simulink model "lab1"  (R2018a)
settings: Solver=ode45  StartTime=0.0  StopTime=5.0  RelTol=1e-3
libraries: powerlib x1
settings Model: Creator=KJ_Fa  LastModifiedBy=KJ_Fa

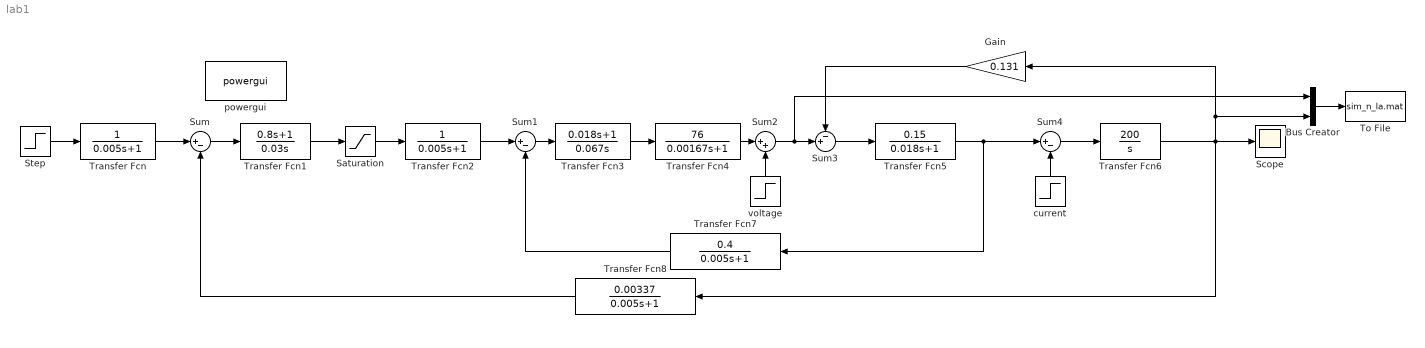
== system lab1 ==
  Bus Creator : BusCreator  Inputs=2
  Gain : Gain  Gain=0.131
  Saturation : Saturate  UpperLimit=8  LowerLimit=-8
  Scope : Scope
  Step : Step  Time=0  After=5  SampleTime=0
  Sum : Sum  Inputs=|+-
  Sum1 : Sum  Inputs=|+-
  Sum2 : Sum  Inputs=|++
  Sum3 : Sum  Inputs=-+|
  Sum4 : Sum  Inputs=|+-
  To File : ToFile  Filename=sim_n_la.mat  MatrixName=signals
  Transfer Fcn : TransferFcn  Denominator=[0.005 1]
  Transfer Fcn1 : TransferFcn  Numerator=[0.8 1]  Denominator=[0.03 0]
  Transfer Fcn2 : TransferFcn  Denominator=[0.005 1]
  Transfer Fcn3 : TransferFcn  Numerator=[0.018 1]  Denominator=[0.067 0]
  Transfer Fcn4 : TransferFcn  Numerator=[76]  Denominator=[0.00167 1]
  Transfer Fcn5 : TransferFcn  Numerator=[0.15]  Denominator=[0.018 1]
  Transfer Fcn6 : TransferFcn  Numerator=[200]  Denominator=[1 0]
  Transfer Fcn7 : TransferFcn  Numerator=[0.4]  Denominator=[0.005 1]
  Transfer Fcn8 : TransferFcn  Numerator=[0.00337]  Denominator=[0.005 1]
  current : Step  Time=3.5  After=0  SampleTime=0
  powergui : powerlib/powergui  Priority=1  SimulationMode=Continuous  SampleTime=50e-6  frequency=60  Iterations=50  frequencyindice=60  Pbase=100e6  ErrMax=1e-4  UnitsV=kV  UnitsW=MW  buscounter=0  FunctionMessages=off  echomessages=off  EnableUseOfTLC=off  CurrentSourceSwitches=off  DisableSnubberDevices=off  DisableRonSwitches=off  DisableVfSwitches=off  DisplayEquations=off  SolverType=Tustin/Backward Euler (TBE)  Interpol=off  ExternalGateDelay=off  methode=off  Ts=100  x0status=blocks  SPID=on  SwTol=0  HookPort=off  RestoreLinks=warning  ResistiveCurrentMeasurement=off  Frange=[0:2:500]  Ylog=off  Xlog=on  ShowGrid=off  save=off  variable=ZData  structure=0  ZoomFFT=off  StartTime=0.0  cycles=1  DisplayStyle=1  fundamental=60  FreqAxis=off  MaxFrequency=1000  frequencyindicesteady=1  RmsSteady=1  display=off
  voltage : Step  Time=3.5  After=-100  SampleTime=0
  wires:
  Step/1 -> Transfer Fcn/1
  Transfer Fcn/1 -> Sum/1
  Sum/1 -> Transfer Fcn1/1
  Transfer Fcn1/1 -> Saturation/1
  Saturation/1 -> Transfer Fcn2/1
  Transfer Fcn2/1 -> Sum1/1
  Sum1/1 -> Transfer Fcn3/1
  Transfer Fcn3/1 -> Transfer Fcn4/1
  Transfer Fcn4/1 -> Sum2/1
  voltage/1 -> Sum2/2
  Sum3/1 -> Transfer Fcn5/1
  Transfer Fcn5/1 -> Sum4/1, Transfer Fcn7/1
  current/1 -> Sum4/2
  Sum4/1 -> Transfer Fcn6/1
  Transfer Fcn6/1 -> Scope/1, Gain/1, Bus Creator/2, Transfer Fcn8/1
  Transfer Fcn7/1 -> Sum1/2
  Transfer Fcn8/1 -> Sum/2
  Bus Creator/1 -> To File/1
  Sum2/1 -> Bus Creator/1, Sum3/2
  Gain/1 -> Sum3/1
